simulink library "socmemlib"  (R2021a)
settings: Solver=VariableStepAuto  StartTime=0.0  StopTime=10.0  RelTol=1e-3
PreLoadFcn:
  | soc.internal.HWSWMessageTypeDef();
  | hsb.blkcb2.defineTypes;
undefined symbols (not defined in the file or in its folder): BurstRequest2BusObj, gcbh, hsb, m, ReadAccessBusObj, rearb, RegA, sendFifoFreeMsg, soc, WriteAccessBusObj
libraries: socmemlib_internal x59, priv_hsblib_beta2 x34, socsharedlib_internal x2, socqueuelib_internal x1, simulink x1
(part 2 of 5)

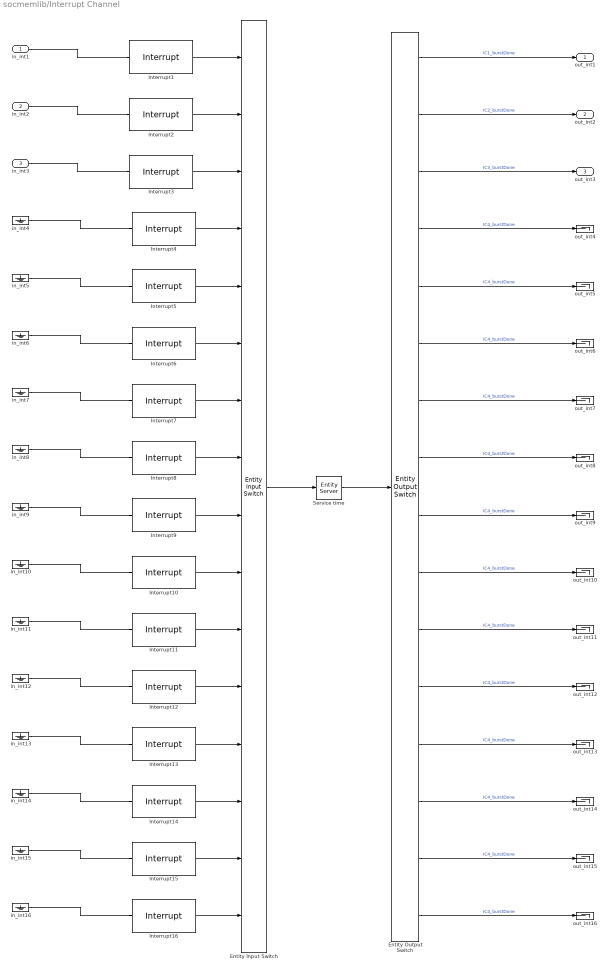
== system socmemlib/Interrupt Channel ==
  in_int1 : Inport
  in_int2 : Inport  Port=2
  in_int3 : Inport  Port=3
  Entity Input Switch : EntityInputSwitch  InputPortMessageModes=m,m,m,m,m,m,m,m,m,m,m,m,m,m,m,m  OutputPortMessageModes=m  NumberInputPorts=16
      settings: InputPortMap=u1,u2,u3,u4,u5,u6,u7,u8,u9,u10,u11,u12,u13,u14,u15,u16
  Entity Output Switch : EntityOutputSwitch  InputPortMessageModes=m  OutputPortMessageModes=m,m,m,m,m,m,m,m,m,m,m,m,m,m,m,m  NumberOutputPorts=16  SwitchingCriterion=From attribute  SwitchAttributeName=custom
      settings: OutputPortMap=o0,o1,o2,o3,o4,o5,o6,o7,o8,o9,o10,o11,o12,o13,o14,o15
  Interrupt1 : socmemlib_internal/Interrupt  Trigger=Rising edge  PortNumber=1
      settings: SourceProductBaseCode=HW
  Interrupt10 : socmemlib_internal/Interrupt  Trigger=None  PortNumber=10
      settings: SourceProductBaseCode=HW
  Interrupt11 : socmemlib_internal/Interrupt  Trigger=None  PortNumber=11
      settings: SourceProductBaseCode=HW
  Interrupt12 : socmemlib_internal/Interrupt  Trigger=None  PortNumber=12
      settings: SourceProductBaseCode=HW
  Interrupt13 : socmemlib_internal/Interrupt  Trigger=None  PortNumber=13
      settings: SourceProductBaseCode=HW
  Interrupt14 : socmemlib_internal/Interrupt  Trigger=None  PortNumber=14
      settings: SourceProductBaseCode=HW
  Interrupt15 : socmemlib_internal/Interrupt  Trigger=None  PortNumber=15
      settings: SourceProductBaseCode=HW
  Interrupt16 : socmemlib_internal/Interrupt  Trigger=None  PortNumber=16
      settings: SourceProductBaseCode=HW
  Interrupt2 : socmemlib_internal/Interrupt  Trigger=Rising edge  PortNumber=2
      settings: SourceProductBaseCode=HW
  Interrupt3 : socmemlib_internal/Interrupt  Trigger=Rising edge  PortNumber=3
      settings: SourceProductBaseCode=HW
  Interrupt4 : socmemlib_internal/Interrupt  Trigger=None  PortNumber=4
      settings: SourceProductBaseCode=HW
  Interrupt5 : socmemlib_internal/Interrupt  Trigger=None  PortNumber=5
      settings: SourceProductBaseCode=HW
  Interrupt6 : socmemlib_internal/Interrupt  Trigger=None  PortNumber=6
      settings: SourceProductBaseCode=HW
  Interrupt7 : socmemlib_internal/Interrupt  Trigger=None  PortNumber=7
      settings: SourceProductBaseCode=HW
  Interrupt8 : socmemlib_internal/Interrupt  Trigger=None  PortNumber=8
      settings: SourceProductBaseCode=HW
  Interrupt9 : socmemlib_internal/Interrupt  Trigger=None  PortNumber=9
      settings: SourceProductBaseCode=HW
  Service time : EntityServer  InputPortMessageModes=m  OutputPortMessageModes=m  Capacity=1  ServiceTimeValue=InterruptProcessingTime
  in_int{4..16} (13 alike) : Ground
  out_int{4..16} (13 alike) : Terminator
  out_int1 : Outport
  out_int2 : Outport  Port=2
  out_int3 : Outport  Port=3
  wires:
  in_int16/1 -> Interrupt16/1
  in_int15/1 -> Interrupt15/1
  in_int14/1 -> Interrupt14/1
  in_int13/1 -> Interrupt13/1
  Interrupt16/1 -> Entity Input Switch/16
  Interrupt15/1 -> Entity Input Switch/15
  Interrupt14/1 -> Entity Input Switch/14
  Interrupt13/1 -> Entity Input Switch/13
  in_int12/1 -> Interrupt12/1
  in_int11/1 -> Interrupt11/1
  in_int10/1 -> Interrupt10/1
  in_int9/1 -> Interrupt9/1
  Interrupt12/1 -> Entity Input Switch/12
  Interrupt11/1 -> Entity Input Switch/11
  Interrupt10/1 -> Entity Input Switch/10
  Interrupt9/1 -> Entity Input Switch/9
  in_int8/1 -> Interrupt8/1
  in_int7/1 -> Interrupt7/1
  in_int6/1 -> Interrupt6/1
  in_int5/1 -> Interrupt5/1
  in_int4/1 -> Interrupt4/1
  in_int3/1 -> Interrupt3/1
  Interrupt8/1 -> Entity Input Switch/8
  Interrupt7/1 -> Entity Input Switch/7
  Interrupt6/1 -> Entity Input Switch/6
  Interrupt5/1 -> Entity Input Switch/5
  Interrupt4/1 -> Entity Input Switch/4
  Interrupt3/1 -> Entity Input Switch/3
  in_int2/1 -> Interrupt2/1
  Interrupt2/1 -> Entity Input Switch/2
  in_int1/1 -> Interrupt1/1
  Interrupt1/1 -> Entity Input Switch/1
  Entity Output Switch/16 -> out_int16/1  "IC4_burstDone"
  Entity Output Switch/15 -> out_int15/1  "IC4_burstDone"
  Entity Output Switch/14 -> out_int14/1  "IC4_burstDone"
  Entity Output Switch/13 -> out_int13/1  "IC4_burstDone"
  Entity Output Switch/12 -> out_int12/1  "IC4_burstDone"
  Entity Output Switch/11 -> out_int11/1  "IC4_burstDone"
  Entity Output Switch/10 -> out_int10/1  "IC4_burstDone"
  Entity Output Switch/9 -> out_int9/1  "IC4_burstDone"
  Entity Output Switch/8 -> out_int8/1  "IC4_burstDone"
  Entity Output Switch/7 -> out_int7/1  "IC4_burstDone"
  Entity Output Switch/6 -> out_int6/1  "IC4_burstDone"
  Entity Output Switch/5 -> out_int5/1  "IC4_burstDone"
  Service time/1 -> Entity Output Switch/1
  Entity Input Switch/1 -> Service time/1
  Entity Output Switch/3 -> out_int3/1  "IC3_burstDone"
  Entity Output Switch/2 -> out_int2/1  "IC2_burstDone"
  Entity Output Switch/4 -> out_int4/1  "IC4_burstDone"
  Entity Output Switch/1 -> out_int1/1  "IC1_burstDone"

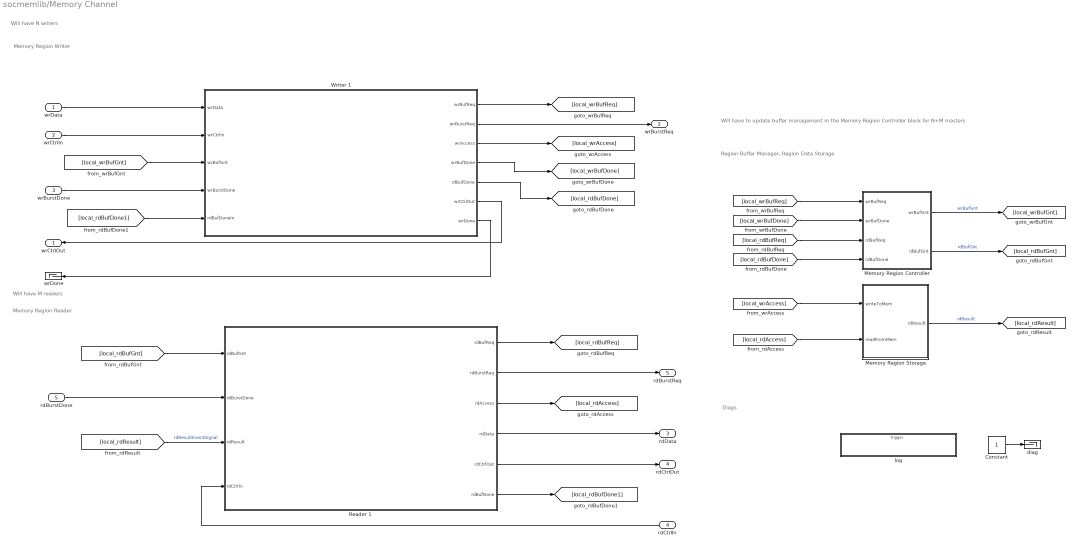
== system socmemlib/Memory Channel ==
  note: Diags
  note: Memory Region Reader
  note: Will have to update buffer management in the
      | Memory Region Controller block for N+M masters
  note: Will have N writers
  note: Region Buffer Manager, Region Data Storage
  note: Memory Region Writer
  note: Will have M readers
  wrData : Inport
  wrCtrlIn : Inport  Port=2  OutDataTypeStr=Bus: StreamM2SBusObj
  wrBurstDone : Inport  Port=3  OutDataTypeStr=Bus: BurstRequest2BusObj
  rdCtrlIn : Inport  Port=4  OutDataTypeStr=Bus: StreamS2MBusObj
  rdBurstDone : Inport  Port=5  OutDataTypeStr=Bus: BurstRequest2BusObj
  Constant : Constant
  Memory Region Controller : Subsystem  mask{RegionBaseAddress=MRBaseAddress, RegionSize=MRRegionSize, NumBuffers=MRNumBuffers, BufSize=MRBufferSize, ReadICDataWidth=blkDP.rsmP.ICDataWidth, WriteICDataWidth=blkDP.wsmP.ICDataWidth, AlignedBufBoundary=blkDP.wsmP.AlignedBufBoundary}
      mask prompts: RegionBaseAddress "Region base byte address"; RegionSize "Region size (bytes)"; NumBuffers "Num buffers"; BufSize "Buf size (bytes)"; ReadICDataWidth "Read interconnect data width (bits)"; WriteICDataWidth "Write interconnect data width (bits)"; AlignedBufBoundary "(aligned buffer boundary)"
      mask help: (internal block) The Memory Region Controller block holds the arbitration and buffer management for a region.
      mask Help: eval('soc.internal.openDoc(''hsb_memoryregioncontrol'')')
  Memory Region Storage : Subsystem  mask{DSMSize=MRRegionSize, MaxWriteSize=blkDP.wsmP.MaxSize, MaxReadSize=blkDP.rsmP.MaxSize, MaximumAccessSize=blkDP.wsmP.MRMaximumAccessSize}
      mask prompts: DSMSize "Data store memory size (bytes)"; MaxWriteSize "Maximum write size (bytes)"; MaxReadSize "Maximum read size (bytes)"; MaximumAccessSize "Maximum access size (bytes)"
      mask help:
      | (internal block) The Memory Region block holds the data store memory for a region.
      | This block holds the memory storage and access interface for a memory region.
      mask Help: eval('soc.internal.openDoc(''hsb_memoryregion'')')
  Reader 1 : Subsystem
  Writer 1 : Subsystem
  diag : Terminator
  log : Subsystem  TreatAsAtomicUnit=on
  wrDone : Terminator
  wrCtrlOut : Outport  OutDataTypeStr=Bus: StreamS2MBusObj  VectorParamsAs1DForOutWhenUnconnected=off
  wrBurstReq : Outport  Port=2  OutDataTypeStr=Bus: BurstRequest2BusObj  VectorParamsAs1DForOutWhenUnconnected=off
  rdData : Outport  Port=3  VectorParamsAs1DForOutWhenUnconnected=off
  rdCtrlOut : Outport  Port=4  OutDataTypeStr=Bus: StreamM2SBusObj  VectorParamsAs1DForOutWhenUnconnected=off
  rdBurstReq : Outport  Port=5  OutDataTypeStr=Bus: BurstRequest2BusObj  VectorParamsAs1DForOutWhenUnconnected=off
  wires:
  Writer 1/5(rdBufDone) -> [local_rdBufDone]
  Reader 1/6(rdBufDone) -> [local_rdBufDone1]
  [local_rdBufDone1] -> Writer 1/5(rdBufDoneIn)
  Writer 1/7(wrDone) -> wrDone/1
  Memory Region Controller/1(wrBufGnt) -> [local_wrBufGnt]  "wrBufGnt"
  Writer 1/2(wrBurstReq) -> wrBurstReq/1
  Writer 1/4(wrBufDone) -> [local_wrBufDone]
  rdCtrlIn/1 -> Reader 1/4(rdCtrlIn)
  Writer 1/1(wrBufReq) -> [local_wrBufReq]
  Reader 1/4(rdData) -> rdData/1
  wrCtrlIn/1 -> Writer 1/2(wrCtrlIn)
  Reader 1/3(rdAccess) -> [local_rdAccess]
  [local_rdResult] -> Reader 1/3(rdResult)  "rdResultEventSignal"
  Constant/1 -> diag/1
  [local_rdBufGnt] -> Reader 1/1(rdBufGnt)
  Reader 1/2(rdBurstReq) -> rdBurstReq/1
  Reader 1/5(rdCtrlOut) -> rdCtrlOut/1
  wrBurstDone/1 -> Writer 1/4(wrBurstDone)
  Writer 1/3(wrAccess) -> [local_wrAccess]
  rdBurstDone/1 -> Reader 1/2(rdBurstDone)
  [local_wrBufDone] -> Memory Region Controller/2(wrBufDone)
  [local_rdBufDone] -> Memory Region Controller/4(rdBufDone)
  Writer 1/6(wrCtrlOut) -> wrCtrlOut/1
  Memory Region Controller/2(rdBufGnt) -> [local_rdBufGnt]  "rdBufGnt"
  Memory Region Storage/1(rdResult) -> [local_rdResult]  "rdResult"
  [local_rdBufReq] -> Memory Region Controller/3(rdBufReq)
  wrData/1 -> Writer 1/1(wrData)
  [local_wrAccess] -> Memory Region Storage/1(writeToMem)
  [local_wrBufGnt] -> Writer 1/3(wrBufGnt)
  [local_wrBufReq] -> Memory Region Controller/1(wrBufReq)
  [local_rdAccess] -> Memory Region Storage/2(readFromMem)
  Reader 1/1(rdBufReq) -> [local_rdBufReq]

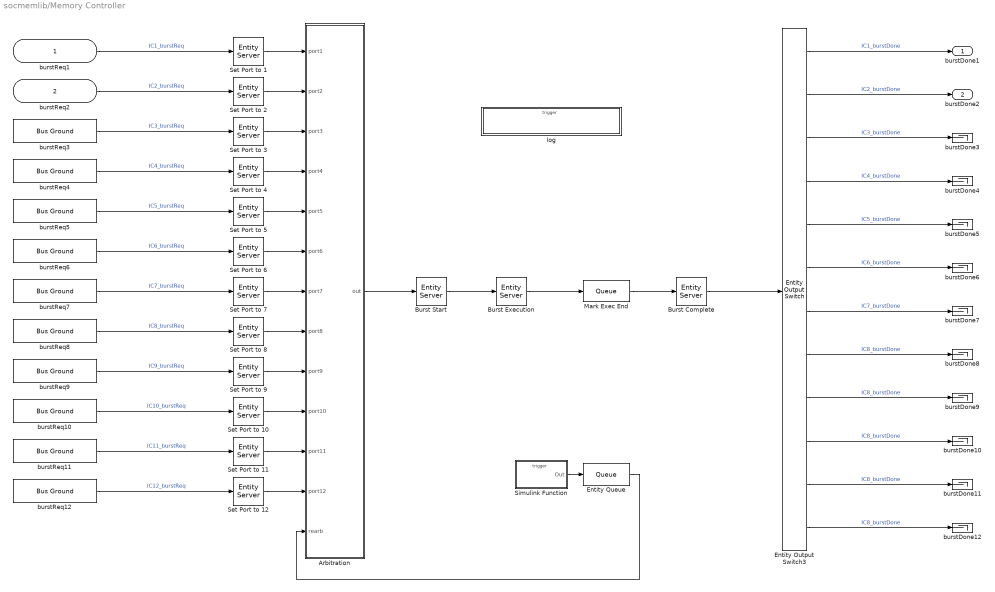
== system socmemlib/Memory Controller ==
  burstReq1 : Inport  OutDataTypeStr=Bus: BurstRequest2BusObj
  burstReq2 : Inport  Port=2  OutDataTypeStr=Bus: BurstRequest2BusObj
  Arbitration : Subsystem  Variant=on  VariantControlMode=label  VariantControl=Variant1  LabelModeActiveChoice=RoundRobin_Variant
  Burst Complete : EntityServer  InputPortMessageModes=m  OutputPortMessageModes=m  Capacity=1  ServiceTimeSource=MATLAB action  ServiceTimeAction=|  ExitAction=|
      ServiceTimeAction=|
      | p.ReqKind = entity.reqKind;
      | p.ControllerClockFrequency = ControllerFrequency;
      | p.ReadLastTransferLatency = ReadLastTransferLatency;
      | p.WriteLastTransferLatency = WriteLastTransferLatency;
      | 
      | dt = hsb.blkcb2.MemoryInterconnectControllerCodegenCb( ...
      |     'BurstCompletionServiceTimeAction',p);
      | 
      | %dt = 20*(1/(ControllerFrequency*1e6));
      ExitAction=|
      | ddinfo = [entity.masterID; entity.reqID; entity.size; entity.addr; 0];
      | ddlogger(entity.port, DDEvent2.BurstComplete, ddinfo);
  Burst Execution : EntityServer  InputPortMessageModes=m  OutputPortMessageModes=m  Capacity=1  ServiceTimeSource=MATLAB action  ServiceTimeAction=|  EntryAction=|  ExitAction=|
      ServiceTimeAction=|
      | p.ReqKind = entity.reqKind;
      | p.ControllerClockFrequency = ControllerFrequency;
      | p.ControllerDataWidth = ControllerDataWidth;
      | p.BurstSize = entity.size;
      | p.BandwidthDerating = BandwidthDerating;
      | p.ReadFirstTransferLatency = ReadFirstTransferLatency;
      | p.WriteFirstTransferLatency = WriteFirstTransferLatency;
      | 
      | dt = hsb.blkcb2.MemoryInterconnectControllerCodegenCb( ...
      |     'BurstExecutionServiceTimeAction',p);
      EntryAction=|
      | ddinfo = [entity.masterID; entity.reqID; entity.size; entity.addr; 0];
      | ddlogger(entity.port, DDEvent2.BurstExecuting, ddinfo);
      ExitAction=|
      | ddinfo = [entity.masterID; entity.reqID; entity.size; entity.addr; 0];
      | ddlogger(entity.port, DDEvent2.BurstDone, ddinfo);
  Burst Start : EntityServer  InputPortMessageModes=m  OutputPortMessageModes=m  Capacity=1  ServiceTimeSource=MATLAB action  ServiceTimeAction=|
      | p.ReqKind = entity.reqKind;
      | p.ControllerClockFrequency = ControllerFrequency;
      | p.ReadFirstTransferLatency = ReadFirstTransferLatency;
      | p.WriteFirstTransferLatency = WriteFirstTransferLatency;
      | 
      | dt = hsb.blkcb2.MemoryInterconnectControllerCodegenCb( ...
      |     'BurstStartServiceTimeAction',p);
  Entity Output Switch3 : EntityOutputSwitch  InputPortMessageModes=m  OutputPortMessageModes=m,m,m,m,m,m,m,m,m,m,m,m  NumberOutputPorts=MAX_NUM_MASTERS  SwitchingCriterion=From attribute  SwitchAttributeName=port
      settings: OutputPortMap=o0,o1,o2,o3,o4,o5,o6,o7,o8,o9,o10,o11
  Entity Queue : Queue  InputPortMessageModes=m  OutputPortMessageModes=m
  Mark Exec End : Queue  InputPortMessageModes=m  OutputPortMessageModes=m  Capacity=1  EntryAction=rearb();
      settings: AttributesFormatString=Capacity=%<Capacity>
  Set Port to 1 : EntityServer  InputPortMessageModes=m  OutputPortMessageModes=m  Capacity=1  ServiceTimeValue=0  EntryAction=|
      | entity.port = 1;
      | entity.state = DDEvent2.BurstRequest;
      | ddinfo = [entity.masterID; entity.reqID; entity.size; entity.addr; 0 ];
      | ddlogger(entity.port, DDEvent2.BurstRequest, ddinfo);
  Set Port to 10 : EntityServer  InputPortMessageModes=m  OutputPortMessageModes=m  Capacity=1  ServiceTimeValue=0  EntryAction=|
      | entity.port = 10;
      | entity.state = DDEvent2.BurstRequest;
      | ddinfo = [entity.masterID; entity.reqID; entity.size; entity.addr; 0 ];
      | ddlogger(entity.port, DDEvent2.BurstRequest, ddinfo);
  Set Port to 11 : EntityServer  InputPortMessageModes=m  OutputPortMessageModes=m  Capacity=1  ServiceTimeValue=0  EntryAction=|
      | entity.port = 11;
      | entity.state = DDEvent2.BurstRequest;
      | ddinfo = [entity.masterID; entity.reqID; entity.size; entity.addr; 0 ];
      | ddlogger(entity.port, DDEvent2.BurstRequest, ddinfo);
  Set Port to 12 : EntityServer  InputPortMessageModes=m  OutputPortMessageModes=m  Capacity=1  ServiceTimeValue=0  EntryAction=|
      | entity.port = 12;
      | entity.state = DDEvent2.BurstRequest;
      | ddinfo = [entity.masterID; entity.reqID; entity.size; entity.addr; 0 ];
      | ddlogger(entity.port, DDEvent2.BurstRequest, ddinfo);
  Set Port to 2 : EntityServer  InputPortMessageModes=m  OutputPortMessageModes=m  Capacity=1  ServiceTimeValue=0  EntryAction=|
      | entity.port = 2;
      | entity.state = DDEvent2.BurstRequest;
      | ddinfo = [entity.masterID; entity.reqID; entity.size; entity.addr; 0 ];
      | ddlogger(entity.port, DDEvent2.BurstRequest, ddinfo);
  Set Port to 3 : EntityServer  InputPortMessageModes=m  OutputPortMessageModes=m  Capacity=1  ServiceTimeValue=0  EntryAction=|
      | entity.port = 3;
      | entity.state = DDEvent2.BurstRequest;
      | ddinfo = [entity.masterID; entity.reqID; entity.size; entity.addr; 0 ];
      | ddlogger(entity.port, DDEvent2.BurstRequest, ddinfo);
  Set Port to 4 : EntityServer  InputPortMessageModes=m  OutputPortMessageModes=m  Capacity=1  ServiceTimeValue=0  EntryAction=|
      | entity.port = 4;
      | entity.state = DDEvent2.BurstRequest;
      | ddinfo = [entity.masterID; entity.reqID; entity.size; entity.addr; 0 ];
      | ddlogger(entity.port, DDEvent2.BurstRequest, ddinfo);
  Set Port to 5 : EntityServer  InputPortMessageModes=m  OutputPortMessageModes=m  Capacity=1  ServiceTimeValue=0  EntryAction=|
      | entity.port = 5;
      | entity.state = DDEvent2.BurstRequest;
      | ddinfo = [entity.masterID; entity.reqID; entity.size; entity.addr; 0 ];
      | ddlogger(entity.port, DDEvent2.BurstRequest, ddinfo);
  Set Port to 6 : EntityServer  InputPortMessageModes=m  OutputPortMessageModes=m  Capacity=1  ServiceTimeValue=0  EntryAction=|
      | entity.port = 6;
      | entity.state = DDEvent2.BurstRequest;
      | ddinfo = [entity.masterID; entity.reqID; entity.size; entity.addr; 0 ];
      | ddlogger(entity.port, DDEvent2.BurstRequest, ddinfo);
  Set Port to 7 : EntityServer  InputPortMessageModes=m  OutputPortMessageModes=m  Capacity=1  ServiceTimeValue=0  EntryAction=|
      | entity.port = 7;
      | entity.state = DDEvent2.BurstRequest;
      | ddinfo = [entity.masterID; entity.reqID; entity.size; entity.addr; 0 ];
      | ddlogger(entity.port, DDEvent2.BurstRequest, ddinfo);
  Set Port to 8 : EntityServer  InputPortMessageModes=m  OutputPortMessageModes=m  Capacity=1  ServiceTimeValue=0  EntryAction=|
      | entity.port = 8;
      | entity.state = DDEvent2.BurstRequest;
      | ddinfo = [entity.masterID; entity.reqID; entity.size; entity.addr; 0 ];
      | ddlogger(entity.port, DDEvent2.BurstRequest, ddinfo);
  Set Port to 9 : EntityServer  InputPortMessageModes=m  OutputPortMessageModes=m  Capacity=1  ServiceTimeValue=0  EntryAction=|
      | entity.port = 9;
      | entity.state = DDEvent2.BurstRequest;
      | ddinfo = [entity.masterID; entity.reqID; entity.size; entity.addr; 0 ];
      | ddlogger(entity.port, DDEvent2.BurstRequest, ddinfo);
  Simulink Function : Subsystem  TreatAsAtomicUnit=on
  burstDone{3..12} (10 alike) : Terminator
  burstReq{3..12} (10 alike) : socmemlib_internal/Bus Ground  OutDataTypeStr=Bus: BurstRequest2BusObj
      settings: SourceProductBaseCode=HW
  log : Subsystem  TreatAsAtomicUnit=on
  burstDone1 : Outport  OutDataTypeStr=Bus: BurstRequest2BusObj  VectorParamsAs1DForOutWhenUnconnected=off
  burstDone2 : Outport  Port=2  OutDataTypeStr=Bus: BurstRequest2BusObj
  wires:
  Entity Output Switch3/12 -> burstDone12/1  "IC8_burstDone"
  Entity Output Switch3/11 -> burstDone11/1  "IC8_burstDone"
  Entity Output Switch3/10 -> burstDone10/1  "IC8_burstDone"
  Entity Output Switch3/9 -> burstDone9/1  "IC8_burstDone"
  Set Port to 12/1 -> Arbitration/12(port12)
  burstReq12/1 -> Set Port to 12/1  "IC12_burstReq"
  Set Port to 11/1 -> Arbitration/11(port11)
  burstReq11/1 -> Set Port to 11/1  "IC11_burstReq"
  Set Port to 10/1 -> Arbitration/10(port10)
  burstReq10/1 -> Set Port to 10/1  "IC10_burstReq"
  Set Port to 9/1 -> Arbitration/9(port9)
  burstReq9/1 -> Set Port to 9/1  "IC9_burstReq"
  Mark Exec End/1 -> Burst Complete/1
  Burst Execution/1 -> Mark Exec End/1
  Arbitration/1(" out") -> Burst Start/1
  Entity Queue/1 -> Arbitration/13(rearb)
  Simulink Function/1(Out) -> Entity Queue/1
  Set Port to 1/1 -> Arbitration/1(port1)
  Set Port to 2/1 -> Arbitration/2("port2 ")
  Set Port to 3/1 -> Arbitration/3("port3 ")
  Set Port to 4/1 -> Arbitration/4("port4 ")
  Set Port to 5/1 -> Arbitration/5("port5 ")
  Set Port to 6/1 -> Arbitration/6("port6 ")
  Set Port to 7/1 -> Arbitration/7("port7 ")
  Set Port to 8/1 -> Arbitration/8("port8 ")
  burstReq6/1 -> Set Port to 6/1  "IC6_burstReq"
  burstReq7/1 -> Set Port to 7/1  "IC7_burstReq"
  Entity Output Switch3/3 -> burstDone3/1  "IC3_burstDone"
  burstReq4/1 -> Set Port to 4/1  "IC4_burstReq"
  Entity Output Switch3/7 -> burstDone7/1  "IC7_burstDone"
  burstReq2/1 -> Set Port to 2/1  "IC2_burstReq"
  Entity Output Switch3/5 -> burstDone5/1  "IC5_burstDone"
  burstReq1/1 -> Set Port to 1/1  "IC1_burstReq"
  Entity Output Switch3/8 -> burstDone8/1  "IC8_burstDone"
  Entity Output Switch3/4 -> burstDone4/1  "IC4_burstDone"
  burstReq3/1 -> Set Port to 3/1  "IC3_burstReq"
  burstReq5/1 -> Set Port to 5/1  "IC5_burstReq"
  Entity Output Switch3/6 -> burstDone6/1  "IC6_burstDone"
  Entity Output Switch3/1 -> burstDone1/1  "IC1_burstDone"
  Entity Output Switch3/2 -> burstDone2/1  "IC2_burstDone"
  burstReq8/1 -> Set Port to 8/1  "IC8_burstReq"
  Burst Complete/1 -> Entity Output Switch3/1
  Burst Start/1 -> Burst Execution/1

== system socmemlib/Memory Traffic Generator ==
  burstDone : Inport  OutDataTypeStr=Bus: BurstRequest2BusObj
  Generate Burst Request : Stateflow chart  TreatAsAtomicUnit=on
  Request Queue with Drops : Subsystem
  burstReq : Outport  OutDataTypeStr=Bus: BurstRequest2BusObj  VectorParamsAs1DForOutWhenUnconnected=off
  wires:
  Generate Burst Request/1(burstReq) -> Request Queue with Drops/1(In1)
  Request Queue with Drops/1(Out1) -> burstReq/1
  burstDone/1 -> Generate Burst Request/1(burstDone)

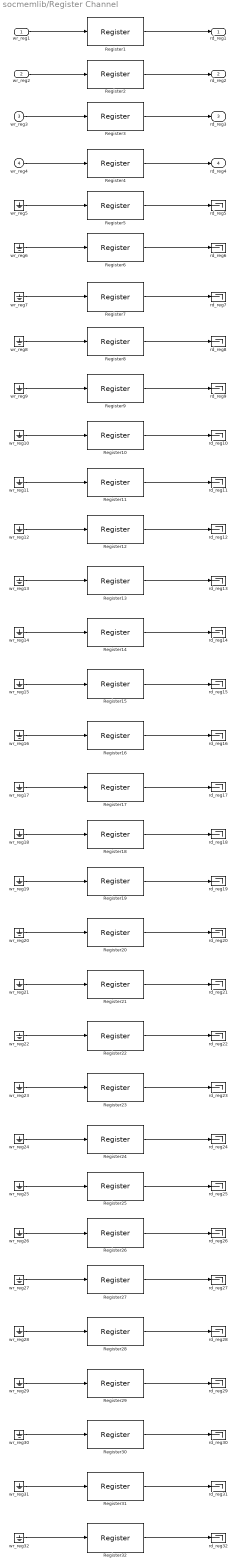
== system socmemlib/Register Channel ==
  wr_reg1 : Inport
  wr_reg2 : Inport  Port=2
  wr_reg3 : Inport  Port=3
  wr_reg4 : Inport  Port=4
  Register1 : socmemlib_internal/Register  Direction=HW to SW  DataTypeStr=uint32  VectorSize=1  SampleTime=-1
      settings: SourceProductBaseCode=HW
  Register{5..32} (28 alike) : socmemlib_internal/Register  Direction=None  DataTypeStr=uint32  VectorSize=1  SampleTime=-1
      settings: SourceProductBaseCode=HW
  Register2 : socmemlib_internal/Register  Direction=HW to SW  DataTypeStr=uint32  VectorSize=1  SampleTime=-1
      settings: SourceProductBaseCode=HW
  Register3 : socmemlib_internal/Register  Direction=SW to HW  DataTypeStr=uint32  VectorSize=1  SampleTime=-1
      settings: SourceProductBaseCode=HW
  Register4 : socmemlib_internal/Register  Direction=SW to HW  DataTypeStr=uint32  VectorSize=1  SampleTime=-1
      settings: SourceProductBaseCode=HW
  rd_reg{5..32} (28 alike) : Terminator
  wr_reg{5..32} (28 alike) : Ground
  rd_reg1 : Outport  VectorParamsAs1DForOutWhenUnconnected=off
  rd_reg2 : Outport  Port=2  VectorParamsAs1DForOutWhenUnconnected=off
  rd_reg3 : Outport  Port=3
  rd_reg4 : Outport  Port=4
  wires:
  Register31/1 -> rd_reg31/1
  wr_reg31/1 -> Register31/1
  wr_reg29/1 -> Register29/1
  wr_reg25/1 -> Register25/1
  wr_reg27/1 -> Register27/1
  Register30/1 -> rd_reg30/1
  Register27/1 -> rd_reg27/1
  wr_reg30/1 -> Register30/1
  Register29/1 -> rd_reg29/1
  Register32/1 -> rd_reg32/1
  wr_reg32/1 -> Register32/1
  Register25/1 -> rd_reg25/1
  Register28/1 -> rd_reg28/1
  wr_reg28/1 -> Register28/1
  Register26/1 -> rd_reg26/1
  wr_reg26/1 -> Register26/1
  Register23/1 -> rd_reg23/1
  wr_reg23/1 -> Register23/1
  wr_reg21/1 -> Register21/1
  wr_reg17/1 -> Register17/1
  wr_reg19/1 -> Register19/1
  Register22/1 -> rd_reg22/1
  Register19/1 -> rd_reg19/1
  wr_reg22/1 -> Register22/1
  Register21/1 -> rd_reg21/1
  Register24/1 -> rd_reg24/1
  wr_reg24/1 -> Register24/1
  Register17/1 -> rd_reg17/1
  Register20/1 -> rd_reg20/1
  wr_reg20/1 -> Register20/1
  Register18/1 -> rd_reg18/1
  wr_reg18/1 -> Register18/1
  wr_reg16/1 -> Register16/1
  Register16/1 -> rd_reg16/1
  wr_reg15/1 -> Register15/1
  Register15/1 -> rd_reg15/1
  wr_reg14/1 -> Register14/1
  Register14/1 -> rd_reg14/1
  wr_reg13/1 -> Register13/1
  Register13/1 -> rd_reg13/1
  wr_reg12/1 -> Register12/1
  Register12/1 -> rd_reg12/1
  wr_reg11/1 -> Register11/1
  Register11/1 -> rd_reg11/1
  wr_reg10/1 -> Register10/1
  Register10/1 -> rd_reg10/1
  wr_reg9/1 -> Register9/1
  Register9/1 -> rd_reg9/1
  wr_reg8/1 -> Register8/1
  Register8/1 -> rd_reg8/1
  wr_reg7/1 -> Register7/1
  Register7/1 -> rd_reg7/1
  wr_reg6/1 -> Register6/1
  Register6/1 -> rd_reg6/1
  wr_reg5/1 -> Register5/1
  Register5/1 -> rd_reg5/1
  wr_reg4/1 -> Register4/1
  Register4/1 -> rd_reg4/1
  Register3/1 -> rd_reg3/1
  wr_reg3/1 -> Register3/1
  Register2/1 -> rd_reg2/1
  wr_reg2/1 -> Register2/1
  Register1/1 -> rd_reg1/1
  wr_reg1/1 -> Register1/1

== system socmemlib/IP Core Register Read/Variant ==
  CODEGEN : Subsystem  VariantControl=(codegen)
  SIM : Subsystem  VariantControl=(sim)
  " Data" : Outport  VectorParamsAs1DForOutWhenUnconnected=off

== system socmemlib/Memory Channel/Memory Region Controller ==
  wrBufReq : Inport
  wrBufDone : Inport  Port=2
  rdBufReq : Inport  Port=3
  rdBufDone : Inport  Port=4
  MemRegionCtrlChart : Stateflow chart  TreatAsAtomicUnit=on
  wrBufGnt : Outport  VectorParamsAs1DForOutWhenUnconnected=off
  rdBufGnt : Outport  Port=2  VectorParamsAs1DForOutWhenUnconnected=off
  wires:
  rdBufReq/1 -> MemRegionCtrlChart/3(rdReq)
  rdBufDone/1 -> MemRegionCtrlChart/4(rdDone)
  MemRegionCtrlChart/2(rdGnt) -> rdBufGnt/1
  MemRegionCtrlChart/1(wrGnt) -> wrBufGnt/1
  wrBufReq/1 -> MemRegionCtrlChart/1(wrReq)
  wrBufDone/1 -> MemRegionCtrlChart/2(wrDone)

== system socmemlib/Memory Channel/Memory Region Storage ==
  writeToMem : Inport
  readFromMem : Inport  Port=2
  Data Store Memory : DataStoreMemory  DataStoreName=MemRegionDataStore  ShowAdditionalParam=off  OutDataTypeStr=uint8  Dimensions=DSMSize  DataLoggingName=MemRegionDataStore
      settings: DataLoggingNameMode=Custom
  Discrete-Event Chart : Stateflow chart  TreatAsAtomicUnit=on
  rdResult : Outport  VectorParamsAs1DForOutWhenUnconnected=off
  wires:
  Discrete-Event Chart/1(rdResult) -> rdResult/1  "rd_data"
  readFromMem/1 -> Discrete-Event Chart/2(rdFromMem)
  writeToMem/1 -> Discrete-Event Chart/1(wrToMem)

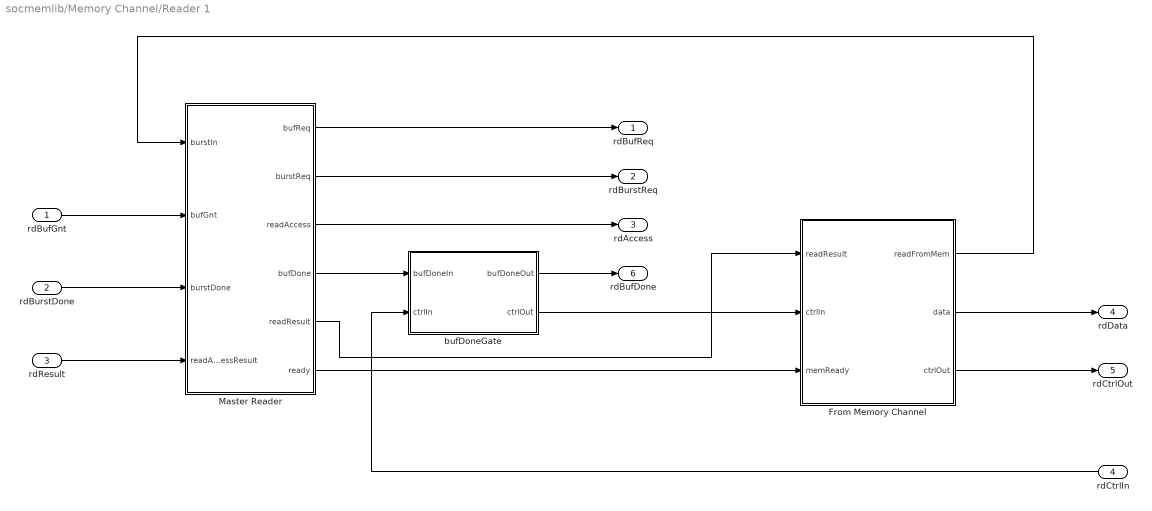
== system socmemlib/Memory Channel/Reader 1 ==
  rdBufGnt : Inport
  rdBurstDone : Inport  Port=2
  rdResult : Inport  Port=3
  rdCtrlIn : Inport  Port=4
  From Memory Channel : Subsystem  Variant=on  VariantControlMode=label  VariantControl=Variant1  LabelModeActiveChoice=StreamingFromMemory_Variant  mask{MasterKind=blkDP.rciP.MasterKind, ChDimensions=blkDP.rciP.ChDimensions, ChType=blkDP.rciP.ChType, ChFrameSampleTime=blkDP.rciP.ChFrameSampleTime, ChBitPacked=blkDP.rciP.ChBitPacked, ChWidth=blkDP.rciP.ChWidth, ChTDATAWidth=blkDP.rciP.ChTDATAWidth, ChTDATAPadWidth=blkDP.rciP.ChTDATAPadWidth, ChCompLength=blkDP.rciP.ChCompLength, ChCompBitRanges=blkDP.rciP.ChCompBitRanges, ChContainerType=blkDP.rciP.ChContainerType, BurstSize=blkDP.rciP.BurstSize, ChGatherBufferBurstCount=blkDP.rciP.ChGatherBufferBurstCount, ChGatherCount=blkDP.rciP.ChGatherCount, ChGatherBufferSize=blkDP.rciP.ChGatherBufferSize, ChFrameGatherBufferSize=blkDP.rciP.ChFrameGatherBufferSize, ChTLASTCount=blkDP.rciP.ChTLASTCount, ChLength=blkDP.rciP.ChLength, EntityInflowTime=blkDP.rciP.EntityInflowTime, InsertInactivePixelClocks=blkDP.rciP.InsertInactivePixelClocks, ActiveVideoLines=blkDP.rciP.ActiveVideoLines, ActivePixelsPerLine=blkDP.rciP.ActivePixelsPerLine, BlankingCount=blkDP.rciP.BlankingCount, PorchCount=blkDP.rciP.PorchCount, InterruptHandlingTime=blkDP.rciP.InterruptHandlingTime, BufferEventID=blkDP.rciP.BufferEventID, NumberOfBuffers=blkDP.rciP.NumberOfBuffers, MaximumBurstSize=blkDP.rciP.MaximumBurstSize, FIFODepth=blkDP.rciP.FIFODepth, FIFOAFullDepth=blkDP.rciP.FIFOAFullDepth}
      mask prompts: MasterKind "(master kind)"; ChDimensions "(dimensions)"; ChType "(ch type)"; ChFrameSampleTime "(sample time)"; ChBitPacked "(columns of data are bit-packed/unpacked)"; ChWidth "(ch width (bits))"; ChTDATAWidth "(ch tdata width (bits))"; ChTDATAPadWidth "(ch tdata padding width (bits))"; ChCompLength "(ch component length)"; ChCompBitRanges "(ch component bit ranges)"; ChContainerType "(ch container type)"; BurstSize "(burst size (bytes))"; ChGatherBufferBurstCount "(ch gather buffer burst count)"; ChGatherCount "(ch gather count)"; ChGatherBufferSize "(ch gather buffer size (bytes))"; ChFrameGatherBufferSize "(ch frame gather buffer size (bytes))"; ChTLASTCount "(ch tlast count)"; ChLength "(ch length)"; EntityInflowTime "(entity inflow time (s))"; InsertInactivePixelClocks "(insert inactive pixel clocks)"; ActiveVideoLines "(active video lines)"; ActivePixelsPerLine "(active pixels per line)"; BlankingCount "(blanking count)"; PorchCount "(porch count)"; InterruptHandlingTime "(interrupt handling time (s))"; BufferEventID "(buffer event ID)"; NumberOfBuffers "(number of buffers)"; MaximumBurstSize "(maximum burst size)"; FIFODepth "(FIFO depth)"; FIFOAFullDepth "(FIFO almost full depth)"
      mask help:
      | A4X from memory logic.
      |
      | The block reads from addressable memory, converts from bytes, and drives a [A4S, A4SV, A4M Write] interface.
      mask DialogControl DerivedParameterGrouprci Prompt: (derived from top-level mask)
      mask DialogControl ChDimensions Tooltip: Dimensions of 'data' signal.
      mask DialogControl ChType Tooltip: Datatype of 'data' signal.
      mask DialogControl ChFrameSampleTime Tooltip: Sample time of 'data' signal. (For frames, it is the full frame time.)
      mask DialogControl ChBitPacked Tooltip:
      | Treat last dimension as channel or pixel data that is packed going to memory.
      | For example, 8bit RGB can be represented as [1x3] in Simulink and packed into
      | 32bit TDATA for the memory interconnect.
      mask DialogControl ChWidth Tooltip: Bit width of 'data' signal.
      mask DialogControl ChTDATAWidth Tooltip: Bit width of 'data' signal implementation. AXI constrains data to certain widths. For example, a 24 bit 'data' signal is placed on a 32 bit datapath in hardware.
      mask DialogControl ChTDATAPadWidth Tooltip:
      | It applies when packing bits for the memory datapath. It specifies the number of bits of
      | padding needed to get to a standard sized container.
      mask DialogControl ChCompLength Tooltip:
      | It applies when packing bits for the memory datapath. It specifies the number of
      | channel components that are bit-packed into TDATA. It is the size of
      | the last dimension.
      mask DialogControl ChCompBitRanges Tooltip:
      | It applies when packing bits for the memory datapath. It specifies the bit locations
      | of the individual channel components that are bit-packed into TDATA.
      mask DialogControl ChContainerType Tooltip: Datatype which holds the 'ChTDATAWidth' bits.
      mask DialogControl BurstSize Tooltip: Size of a burst in bytes. It is derived from 'BurstLength' and 'ChContainerType'.
      mask DialogControl ChGatherBufferBurstCount Tooltip:
      | Number of bursts (always an integer) held in a gather buffer.
      | If 'data' dimensions are less than a burst, the gather buffer gathers 'data' transfers until it has a burst.
      | If 'data' dimensions are greater than a burst, the gather buffer fills with one transfer and can represent >1 burst.
      mask DialogControl ChGatherCount Tooltip: Number of 'data' transfers needed to gather a full burst.
      mask DialogControl ChGatherBufferSize Tooltip: Size of gather buffer in bytes. It is 'ChGatherBurstCount' times 'BurstSize'.
      mask DialogControl ChFrameGatherBufferSize Tooltip: Number of bytes that each transfer of 'data' signal adds to the internal gather buffer.
      mask DialogControl ChTLASTCount Tooltip: Count of 'data' transfers that comprise a memory region buffer. TLAST marks the end of a buffer.
      mask DialogControl ChLength Tooltip: Number of scalar data in each 'data' transfer. It is the product of 'ChDimensions'.
      mask DialogControl EntityInflowTime Tooltip:
      | Pacing of bursts to memory. It only applies if a 'data' transfer is greater than a burst.
      | If 'data' is less than a burst, time has already been spent gathering the buffer. In this case, the pacing time is 0.
      mask DialogControl InsertInactivePixelClocks Tooltip: Number of active lines in the video frame
      mask DialogControl ActiveVideoLines Tooltip: Number of active lines in the video frame
      mask DialogControl ActivePixelsPerLine Tooltip: Number of active pixels per line in the video frame
      mask DialogControl BlankingCount Tooltip: Number of inactive lines in the video frame
      mask DialogControl PorchCount Tooltip: Number of inactive pixels per line in the video frame
      mask DialogControl MaximumBurstSize Tooltip: Maximum burst size (in bytes) to memory, a fixed constant for the system.
  Master Reader : Subsystem  VariantControl=BlockMaster_Variant  mask{MasterID=blkDP.rmicP.MasterID, MasterKind=blkDP.rmicP.MasterKind, EntityInflowQueueCapacity=blkDP.rmicP.EntityInflowQueueCapacity, EntityInflowTime=blkDP.rmicP.EntityInflowTime, AccessTransactionType=ReadAccessBusObj, FIFODepth=blkDP.rmicP.FIFODepth, FIFOAFullDepth=blkDP.rmicP.FIFOAFullDepth, BufferLengthInBursts=blkDP.rmicP.BufferLengthInBursts, ICClockFrequency=blkDP.rmicP.ICClockFrequency, ICDataWidth=blkDP.rmicP.ICDataWidth}
      mask prompts: MasterID "(master id)"; MasterKind "(master kind)"; EntityInflowQueueCapacity "(inflow queue capacity)"; EntityInflowTime "(entity inflow time)"; AccessTransactionType "(access transaction type)"; FIFODepth "(FIFO depth)"; FIFOAFullDepth "(FIFO almost full depth)"; BufferLengthInBursts "(Buffer length in bursts)"; ICClockFrequency "(interconnect clock frequency)"; ICDataWidth "(interconnect data width)"
      mask help:
      | Generic reader mem channel logic
      |
      | The block takes read access transactions from the protocol s/m and models execution of those transactions.
      mask DialogControl DerivedParameterGrouprmic Prompt: (derived from top-level mask)
  bufDoneGate : Subsystem  Variant=on  VariantControlMode=label  VariantControl=Variant1  LabelModeActiveChoice=passthrough
  rdBufReq : Outport  VectorParamsAs1DForOutWhenUnconnected=off
  rdBurstReq : Outport  Port=2  VectorParamsAs1DForOutWhenUnconnected=off
  rdAccess : Outport  Port=3  VectorParamsAs1DForOutWhenUnconnected=off
  rdData : Outport  Port=4  VectorParamsAs1DForOutWhenUnconnected=off
  rdCtrlOut : Outport  Port=5  VectorParamsAs1DForOutWhenUnconnected=off
  rdBufDone : Outport  Port=6  VectorParamsAs1DForOutWhenUnconnected=off
  wires:
  From Memory Channel/3(" ctrlOut") -> rdCtrlOut/1
  From Memory Channel/2(" data") -> rdData/1
  bufDoneGate/2(" ctrlOut") -> From Memory Channel/2("ctrlIn ")
  bufDoneGate/1(" bufDoneOut") -> rdBufDone/1
  rdCtrlIn/1 -> bufDoneGate/2("ctrlIn ")
  Master Reader/4(bufDone) -> bufDoneGate/1("bufDoneIn ")
  Master Reader/2(burstReq) -> rdBurstReq/1
  Master Reader/3(readAccess) -> rdAccess/1
  rdResult/1 -> Master Reader/4(readAccessResult)
  Master Reader/6(ready) -> From Memory Channel/3(memReady)
  rdBurstDone/1 -> Master Reader/3(burstDone)
  Master Reader/1(bufReq) -> rdBufReq/1
  rdBufGnt/1 -> Master Reader/2(bufGnt)
  Master Reader/5(readResult) -> From Memory Channel/1("readResult ")
  From Memory Channel/1(" readFromMem") -> Master Reader/1(burstIn)

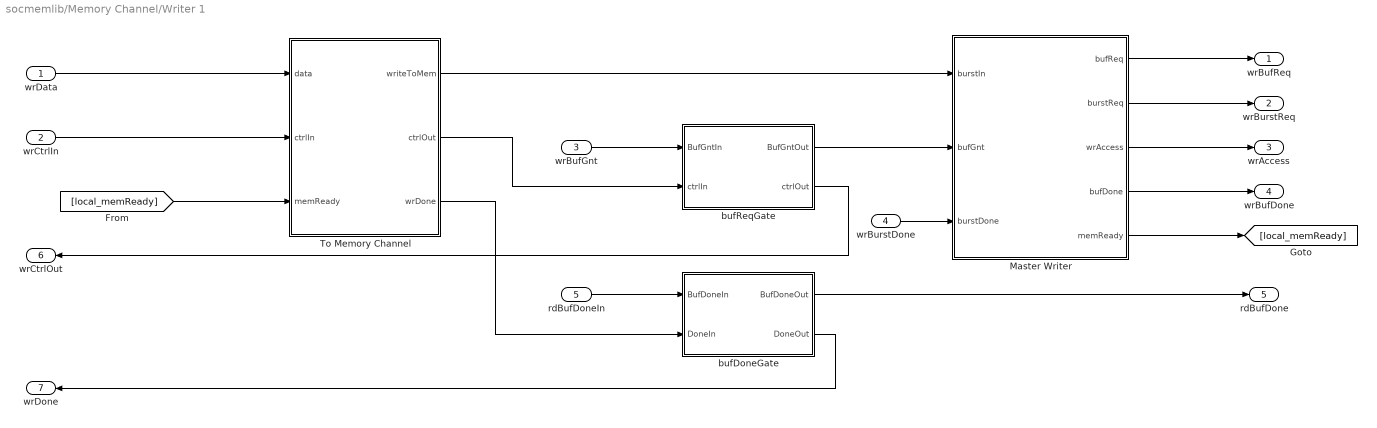
== system socmemlib/Memory Channel/Writer 1 ==
  wrData : Inport
  wrCtrlIn : Inport  Port=2
  wrBufGnt : Inport  Port=3
  wrBurstDone : Inport  Port=4
  rdBufDoneIn : Inport  Port=5
  Master Writer : Subsystem  VariantControl=BlockMaster_Variant  mask{MasterID=blkDP.wmicP.MasterID, MasterKind=blkDP.wmicP.MasterKind, EntityInflowQueueCapacity=blkDP.wmicP.EntityInflowQueueCapacity, EntityInflowTime=blkDP.wmicP.EntityInflowTime, AccessTransactionType=WriteAccessBusObj, FIFODepth=blkDP.wmicP.FIFODepth, FIFOAFullDepth=blkDP.wmicP.FIFOAFullDepth, BufferLengthInBursts=blkDP.wmicP.BufferLengthInBursts, ICClockFrequency=blkDP.wmicP.ICClockFrequency, ICDataWidth=blkDP.wmicP.ICDataWidth}
      mask prompts: MasterID "(master id)"; MasterKind "(master kind)"; EntityInflowQueueCapacity "(inflow queue capacity)"; EntityInflowTime "(entity inflow time)"; AccessTransactionType "(access transaction type)"; FIFODepth "(FIFO depth)"; FIFOAFullDepth "(FIFO almost full depth)"; BufferLengthInBursts "(Buffer length in bursts)"; ICClockFrequency "(interconnect clock frequency)"; ICDataWidth "(interconnect data width)"
      mask help:
      | Generic writer mem channel logic
      |
      | The block takes write access transactions from the protocol s/m and models execution of those transactions.
      mask DialogControl DerivedParameterGroupwmic Prompt: (derived from top-level mask)
  To Memory Channel : Subsystem  Variant=on  VariantControlMode=label  VariantControl=Variant1  LabelModeActiveChoice=StreamingToMemory_Variant  mask{MasterKind=blkDP.wciP.MasterKind, ChDimensions=blkDP.wciP.ChDimensions, ChType=blkDP.wciP.ChType, ChFrameSampleTime=blkDP.wciP.ChFrameSampleTime, ChBitPacked=blkDP.wciP.ChBitPacked, ChWidth=blkDP.wciP.ChWidth, ChTDATAWidth=blkDP.wciP.ChTDATAWidth, ChTDATAPadWidth=blkDP.wciP.ChTDATAPadWidth, ChCompLength=blkDP.wciP.ChCompLength, ChCompBitRanges=blkDP.wciP.ChCompBitRanges, ChContainerType=blkDP.wciP.ChContainerType, BurstSize=blkDP.wciP.BurstSize, ChGatherBufferBurstCount=blkDP.wciP.ChGatherBufferBurstCount, ChGatherCount=blkDP.wciP.ChGatherCount, ChGatherBufferSize=blkDP.wciP.ChGatherBufferSize, ChFrameGatherBufferSize=blkDP.wciP.ChFrameGatherBufferSize, ChTLASTCount=blkDP.wciP.ChTLASTCount, ChLength=blkDP.wciP.ChLength, EntityInflowTime=blkDP.wciP.EntityInflowTime, InterruptHandlingTime=blkDP.wciP.InterruptHandlingTime, BufferEventID=blkDP.wciP.BufferEventID, NumberOfBuffers=blkDP.wciP.NumberOfBuffers, MaximumBurstSize=blkDP.wciP.MaximumBurstSize}
      mask prompts: MasterKind "(master kind)"; ChDimensions "(dimensions)"; ChType "(ch type)"; ChFrameSampleTime "(sample time)"; ChBitPacked "(columns of data are bit-packed/unpacked)"; ChWidth "(ch width (bits))"; ChTDATAWidth "(ch tdata width (bits))"; ChTDATAPadWidth "(ch tdata padding width (bits))"; ChCompLength "(ch component length)"; ChCompBitRanges "(ch component bit ranges)"; ChContainerType "(ch container type)"; BurstSize "(burst size (bytes))"; ChGatherBufferBurstCount "(ch gather buffer burst count)"; ChGatherCount "(ch gather count)"; ChGatherBufferSize "(ch gather buffer size (bytes))"; ChFrameGatherBufferSize "(ch frame gather buffer size (bytes))"; ChTLASTCount "(ch tlast count)"; ChLength "(ch length)"; EntityInflowTime "(entity inflow time (s))"; InterruptHandlingTime "(interrupt handling time (s))"; BufferEventID "(buffer event ID)"; NumberOfBuffers "(number of buffers)"; MaximumBurstSize "(maximum burst size)"
      mask help:
      | A4X to memory state machine.
      |
      | The block takes [A4S, A4SV, A4M Write], converts it to bytes, and writes it to addressable memory.
      mask DialogControl DerivedParameterGroupwci Prompt: (derived from top-level mask)
      mask DialogControl ChDimensions Tooltip: Dimensions of 'data' signal.
      mask DialogControl ChType Tooltip: Datatype of 'data' signal.
      mask DialogControl ChFrameSampleTime Tooltip: Sample time of 'data' signal. (For frames, it is the full frame time.)
      mask DialogControl ChBitPacked Tooltip:
      | Treat last dimension as channel or pixel data that is packed going to memory.
      | For example, 8bit RGB can be represented as [1x3] in Simulink and packed into
      | 32bit TDATA for the memory interconnect.
      mask DialogControl ChWidth Tooltip: Bit width of 'data' signal.
      mask DialogControl ChTDATAWidth Tooltip: Bit width of 'data' signal implementation. AXI constrains data to certain widths. For example, a 24 bit 'data' signal is placed on a 32 bit datapath in hardware.
      mask DialogControl ChTDATAPadWidth Tooltip:
      | It applies when packing bits for the memory datapath. It specifies the number of bits of
      | padding needed to get to a standard sized container.
      mask DialogControl ChCompLength Tooltip:
      | It applies when packing bits for the memory datapath. It specifies the number of
      | channel components that are bit-packed into TDATA. It is the size of
      | the last dimension.
      mask DialogControl ChCompBitRanges Tooltip:
      | It applies when packing bits for the memory datapath. It specifies the bit locations
      | of the individual channel components that are bit-packed into TDATA.
      mask DialogControl ChContainerType Tooltip: Datatype which holds the 'ChTDATAWidth' bits.
      mask DialogControl BurstSize Tooltip: Size of a burst in bytes. It is derived from 'BurstLength' and 'ChContainerType'.
      mask DialogControl ChGatherBufferBurstCount Tooltip:
      | Number of bursts (always an integer) held in a gather buffer.
      | If 'data' dimensions are less than a burst, the gather buffer gathers 'data' transfers until it has a burst.
      | If 'data' dimensions are greater than a burst, the gather buffer fills with one transfer and can represent >1 burst.
      mask DialogControl ChGatherCount Tooltip: Number of 'data' transfers needed to gather a full burst.
      mask DialogControl ChGatherBufferSize Tooltip: Size of gather buffer in bytes. It is 'ChGatherBurstCount' times 'BurstSize'.
      mask DialogControl ChFrameGatherBufferSize Tooltip: Number of bytes that each transfer of 'data' signal adds to the internal gather buffer.
      mask DialogControl ChTLASTCount Tooltip: Count of 'data' transfers that comprise a memory region buffer. TLAST marks the end of a buffer.
      mask DialogControl ChLength Tooltip: Number of scalar data in each 'data' transfer. It is the product of 'ChDimensions'.
      mask DialogControl EntityInflowTime Tooltip:
      | Pacing of bursts to memory. It only applies if a 'data' transfer is greater than a burst.
      | If 'data' is less than a burst, time has already been spent gathering the buffer. In this case, the pacing time is 0.
      mask DialogControl MaximumBurstSize Tooltip: Maximum burst size (in bytes) to memory, a fixed constant for the system.
  bufDoneGate : Subsystem  Variant=on  VariantControlMode=label  VariantControl=Variant1  LabelModeActiveChoice=passthrough
  bufReqGate : Subsystem  Variant=on  VariantControlMode=label  VariantControl=Variant1  LabelModeActiveChoice=passthrough
  wrBufReq : Outport  VectorParamsAs1DForOutWhenUnconnected=off
  wrBurstReq : Outport  Port=2  VectorParamsAs1DForOutWhenUnconnected=off
  wrAccess : Outport  Port=3  VectorParamsAs1DForOutWhenUnconnected=off
  wrBufDone : Outport  Port=4  VectorParamsAs1DForOutWhenUnconnected=off
  rdBufDone : Outport  Port=5  VectorParamsAs1DForOutWhenUnconnected=off
  wrCtrlOut : Outport  Port=6  VectorParamsAs1DForOutWhenUnconnected=off
  wrDone : Outport  Port=7
  wires:
  bufDoneGate/1(" BufDoneOut") -> rdBufDone/1
  rdBufDoneIn/1 -> bufDoneGate/1("BufDoneIn ")
  To Memory Channel/3(wrDone) -> bufDoneGate/2("DoneIn ")
  wrBufGnt/1 -> bufReqGate/1("BufGntIn ")
  bufReqGate/1(" BufGntOut") -> Master Writer/2(bufGnt)
  bufReqGate/2(" ctrlOut") -> wrCtrlOut/1
  To Memory Channel/2(" ctrlOut") -> bufReqGate/2("ctrlIn ")
  bufDoneGate/2(" DoneOut") -> wrDone/1
  Master Writer/4(bufDone) -> wrBufDone/1
  Master Writer/3(wrAccess) -> wrAccess/1
  [local_memReady] -> To Memory Channel/3(memReady)
  wrCtrlIn/1 -> To Memory Channel/2("ctrlIn ")
  Master Writer/2(burstReq) -> wrBurstReq/1
  wrBurstDone/1 -> Master Writer/3(burstDone)
  To Memory Channel/1(" writeToMem") -> Master Writer/1(burstIn)
  Master Writer/1(bufReq) -> wrBufReq/1
  Master Writer/5(memReady) -> [local_memReady]
  wrData/1 -> To Memory Channel/1("data ")

== system socmemlib/Memory Channel/log ==
  ddlogger : TriggerPort  TriggerType=function-call  IsSimulinkFunction=on  FunctionName=ddlogger  FunctionVisibility=scoped  VariantControl=(inherit)
  Constant : Constant
  Constant1 : Constant  Value=2
  MATLAB Function : MATLAB Function  TreatAsAtomicUnit=on  VariantControl=DebugLevel2_Variant
  Reader : priv_hsblib_beta2/MemCh Diag Sigs L2  SystemSampleTime=-1  VariantActivationTime=update diagram  Latency=0  AutoFrameSizeCalculation=off
      settings: SourceProductBaseCode=HW
  Writer : priv_hsblib_beta2/MemCh Diag Sigs L2  SystemSampleTime=-1  VariantActivationTime=update diagram  Latency=0  AutoFrameSizeCalculation=off
      settings: SourceProductBaseCode=HW
  mid : ArgIn  DisableCoverage=on  ArgumentName=mid
  event : ArgIn  Port=2  OutDataTypeStr=Enum: DDEvent2  ArgumentName=event
  info : ArgIn  Port=3  PortDimensions=5  ArgumentName=info
  wires:
  mid/1 -> MATLAB Function/1(mID)
  event/1 -> MATLAB Function/2(event)
  info/1 -> MATLAB Function/3(info)
  Constant/1 -> Writer/2
  Constant1/1 -> Reader/2
  MATLAB Function/1(ddOut) -> Writer/1, Reader/1

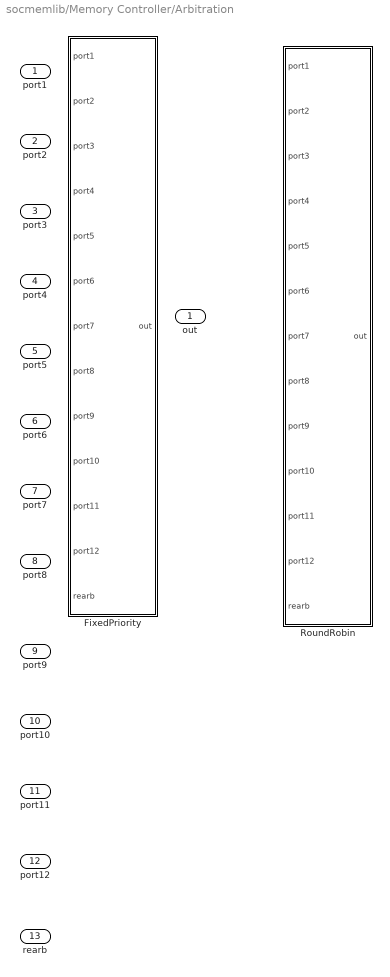
== system socmemlib/Memory Controller/Arbitration ==
  port1 : Inport
  "port2 " : Inport  Port=2
  "port3 " : Inport  Port=3
  "port4 " : Inport  Port=4
  "port5 " : Inport  Port=5
  "port6 " : Inport  Port=6
  "port7 " : Inport  Port=7
  "port8 " : Inport  Port=8
  port9 : Inport  Port=9
  port10 : Inport  Port=10
  port11 : Inport  Port=11
  port12 : Inport  Port=12
  rearb : Inport  Port=13
  FixedPriority : Subsystem  VariantControl=FixedPriority_Variant
  RoundRobin : Subsystem  VariantControl=RoundRobin_Variant
  " out" : Outport  VectorParamsAs1DForOutWhenUnconnected=off

== system socmemlib/Memory Controller/Simulink Function ==
  rearb : TriggerPort  TriggerType=function-call  IsSimulinkFunction=on  FunctionName=rearb  FunctionVisibility=scoped  VariantControl=Variant
  Constant : Constant
  Message Send : Send  OutputPortMessageModes=m
  Out : Outport  VectorParamsAs1DForOutWhenUnconnected=off
  wires:
  Constant/1 -> Message Send/1
  Message Send/1 -> Out/1

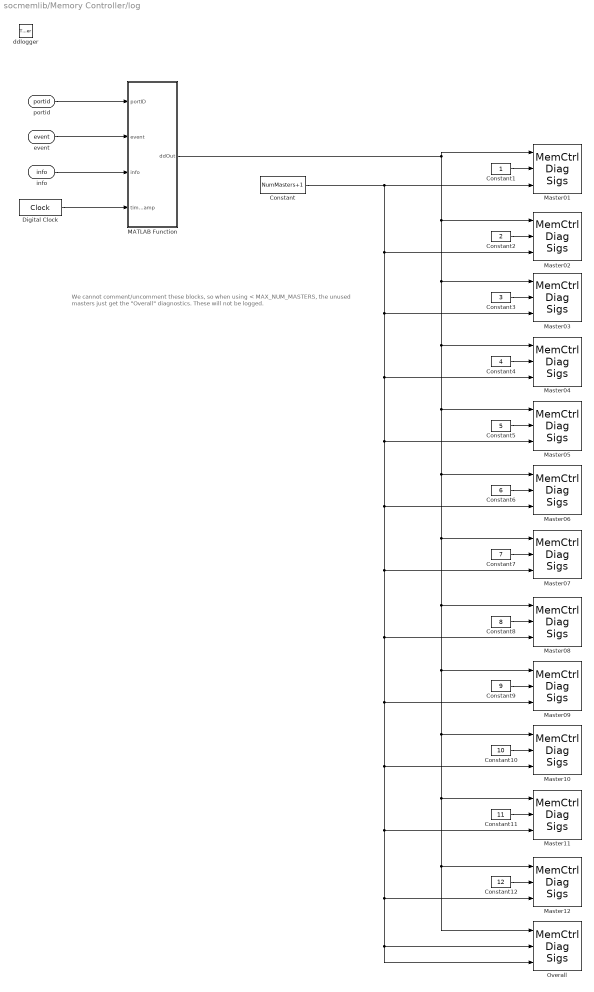
== system socmemlib/Memory Controller/log ==
  note: We cannot comment/uncomment these blocks, so when
      | using < MAX_NUM_MASTERS, the unused masters just
      | get the "Overall" diagnostics. These will not be logged.
  ddlogger : TriggerPort  TriggerType=function-call  IsSimulinkFunction=on  FunctionName=ddlogger  FunctionVisibility=scoped  VariantControl=(inherit)
  Constant : Constant  Value=NumMasters+1
  Constant1 : Constant
  Constant10 : Constant  Value=10
  Constant11 : Constant  Value=11
  Constant12 : Constant  Value=12
  Constant2 : Constant  Value=2
  Constant3 : Constant  Value=3
  Constant4 : Constant  Value=4
  Constant5 : Constant  Value=5
  Constant6 : Constant  Value=6
  Constant7 : Constant  Value=7
  Constant8 : Constant  Value=8
  Constant9 : Constant  Value=9
  Digital Clock : DigitalClock  SampleTime=-1
  MATLAB Function : MATLAB Function  TreatAsAtomicUnit=on
  Master01 : priv_hsblib_beta2/MemCtrl Diag Sigs  SystemSampleTime=-1  VariantActivationTime=update diagram  Latency=0  AutoFrameSizeCalculation=off
      settings: SourceProductBaseCode=HW
  Master02 : priv_hsblib_beta2/MemCtrl Diag Sigs  SystemSampleTime=-1  VariantActivationTime=update diagram  Latency=0  AutoFrameSizeCalculation=off
      settings: SourceProductBaseCode=HW
  Master03 : priv_hsblib_beta2/MemCtrl Diag Sigs  SystemSampleTime=-1  VariantActivationTime=update diagram  Latency=0  AutoFrameSizeCalculation=off
      settings: SourceProductBaseCode=HW
  Master04 : priv_hsblib_beta2/MemCtrl Diag Sigs  SystemSampleTime=-1  VariantActivationTime=update diagram  Latency=0  AutoFrameSizeCalculation=off
      settings: SourceProductBaseCode=HW
  Master05 : priv_hsblib_beta2/MemCtrl Diag Sigs  SystemSampleTime=-1  VariantActivationTime=update diagram  Latency=0  AutoFrameSizeCalculation=off
      settings: SourceProductBaseCode=HW
  Master06 : priv_hsblib_beta2/MemCtrl Diag Sigs  SystemSampleTime=-1  VariantActivationTime=update diagram  Latency=0  AutoFrameSizeCalculation=off
      settings: SourceProductBaseCode=HW
  Master07 : priv_hsblib_beta2/MemCtrl Diag Sigs  SystemSampleTime=-1  VariantActivationTime=update diagram  Latency=0  AutoFrameSizeCalculation=off
      settings: SourceProductBaseCode=HW
  Master08 : priv_hsblib_beta2/MemCtrl Diag Sigs  SystemSampleTime=-1  VariantActivationTime=update diagram  Latency=0  AutoFrameSizeCalculation=off
      settings: SourceProductBaseCode=HW
  Master09 : priv_hsblib_beta2/MemCtrl Diag Sigs  SystemSampleTime=-1  VariantActivationTime=update diagram  Latency=0  AutoFrameSizeCalculation=off
      settings: SourceProductBaseCode=HW
  Master10 : priv_hsblib_beta2/MemCtrl Diag Sigs  SystemSampleTime=-1  VariantActivationTime=update diagram  Latency=0  AutoFrameSizeCalculation=off
      settings: SourceProductBaseCode=HW
  Master11 : priv_hsblib_beta2/MemCtrl Diag Sigs  SystemSampleTime=-1  VariantActivationTime=update diagram  Latency=0  AutoFrameSizeCalculation=off
      settings: SourceProductBaseCode=HW
  Master12 : priv_hsblib_beta2/MemCtrl Diag Sigs  SystemSampleTime=-1  VariantActivationTime=update diagram  Latency=0  AutoFrameSizeCalculation=off
      settings: SourceProductBaseCode=HW
  Overall : priv_hsblib_beta2/MemCtrl Diag Sigs  SystemSampleTime=-1  VariantActivationTime=update diagram  Latency=0  AutoFrameSizeCalculation=off
      settings: SourceProductBaseCode=HW
  portid : ArgIn  DisableCoverage=on  ArgumentName=portid
  event : ArgIn  Port=2  OutDataTypeStr=Enum: DDEvent2  ArgumentName=event
  info : ArgIn  Port=3  PortDimensions=5  ArgumentName=info
  wires:
  Digital Clock/1 -> MATLAB Function/4(timestamp)
  info/1 -> MATLAB Function/3(info)
  event/1 -> MATLAB Function/2(event)
  portid/1 -> MATLAB Function/1(portID)
  Constant9/1 -> Master09/2
  Constant5/1 -> Master05/2
  Constant6/1 -> Master06/2
  Constant12/1 -> Master12/2
  Constant8/1 -> Master08/2
  Constant2/1 -> Master02/2
  MATLAB Function/1(ddOut) -> Master02/1, Master03/1, Master04/1, Master05/1, Master06/1, Master07/1, Master08/1, Master09/1, Master10/1, Master11/1, Master12/1, Overall/1, Master01/1
  Constant3/1 -> Master03/2
  Constant4/1 -> Master04/2
  Constant/1 -> Master01/3, Master02/3, Master03/3, Master04/3, Master05/3, Master06/3, Master07/3, Master08/3, Master09/3, Master10/3, Master11/3, Master12/3, Overall/2, Overall/3
  Constant7/1 -> Master07/2
  Constant10/1 -> Master10/2
  Constant11/1 -> Master11/2
  Constant1/1 -> Master01/2

== system socmemlib/Memory Traffic Generator/Request Queue with Drops ==
  In1 : Inport
  Assert : Assertion  AssertionFailFcn=disp(['Memory Traffic Generator ' gcb ' dropped a burst done.'])  StopWhenAssertionFail=off
  Compare To Zero1 : simulink/Logic and Bit Operations/Compare To Zero  relop===  OutDataTypeStr=boolean  ZeroCross=off
  Entity Terminator1 : EntityTerminator  InputPortMessageModes=m  EntryAction=|
      | o = entity(5);
      | extractOverflow(o);
  FIFO with Drops : Subsystem  mask{FIFOTransactionType=BurstRequest2BusObj, FIFODepth=10, FIFOAFullDepth=10}
      mask prompts: FIFOTransactionType "FIFO transaction type"; FIFODepth "FIFO depth (num bursts)"; FIFOAFullDepth "FIFO almost full depth (num bursts)"
  Simulink Function : Subsystem  TreatAsAtomicUnit=on
  Out1 : Outport  VectorParamsAs1DForOutWhenUnconnected=off
  wires:
  Simulink Function/1(overrun) -> Compare To Zero1/1
  Compare To Zero1/1 -> Assert/1
  FIFO with Drops/2(fifoStatusMsg) -> Entity Terminator1/1
  FIFO with Drops/1(transactionOut) -> Out1/1
  In1/1 -> FIFO with Drops/1(transactionIn)

== system socmemlib/IP Core Register Read/Variant/CODEGEN ==
  Constant : Constant  Value=RegA  OutDataTypeStr=uint16  SampleTime=-1
  " Data" : Outport  VectorParamsAs1DForOutWhenUnconnected=off
  wires:
  Constant/1 -> " Data"/1
